simulink model "Ejercicio_2_DB"  (R2019b)
settings: Solver=VariableStepAuto  StartTime=0.0  StopTime=6  MinStep=0.001  RelTol=1e-3
values from neighbouring files (symbols this model uses):
  K = 2.22    [Ejercicio_2.m]
  Kt = K-1    (= 1.22)    [Ejercicio_2.m]
libraries: simulink x1
settings Model: Creator=54115  LastModifiedBy=54115

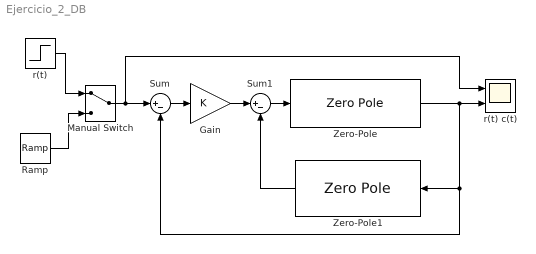
== system Ejercicio_2_DB ==
  Gain : Gain  Gain=K
  Manual Switch : ManualSwitch
  Ramp : simulink/Sources/Ramp  slope=1  start=0  InitialOutput=0
  Sum : Sum  Inputs=|+-
  Sum1 : Sum  Inputs=|+-
  Zero-Pole : ZeroPole  Zeros=[]  Poles=[0 -1 -10]  Gain=[10]
  Zero-Pole1 : ZeroPole  Zeros=[0]  Poles=[-100]  Gain=[100*Kt]
  r(t) : Step  Time=0  SampleTime=0
  r(t) c(t) : Scope  NumInputPorts=2
  wires:
  Zero-Pole/1 -> r(t) c(t)/2, Zero-Pole1/1, Sum/2
  Sum1/1 -> Zero-Pole/1
  Gain/1 -> Sum1/1
  Sum/1 -> Gain/1
  Manual Switch/1 -> r(t) c(t)/1, Sum/1
  r(t)/1 -> Manual Switch/1
  Ramp/1 -> Manual Switch/2
  Zero-Pole1/1 -> Sum1/2
